simulink library "LibConfigurableSubsystem"  (R2015b)
settings: Solver=VariableStepAuto  StartTime=0.0  StopTime=10.0  RelTol=1e-3
libraries: LibConfigurableSubsystem x1
settings Model: Creator=LUBO  LastModifiedBy=LUBO

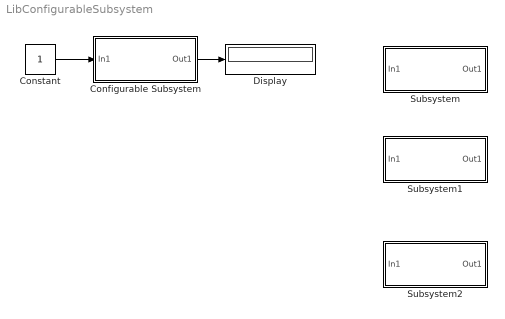
== system LibConfigurableSubsystem ==
  Configurable Subsystem : Subsystem  BlockChoice=Subsystem2
      settings: TemplateBlock=self  MemberBlocks=Subsystem,Subsystem1,Subsystem2
  Constant : Constant
  Display : Display
  Subsystem : Subsystem
  Subsystem1 : Subsystem
  Subsystem2 : Subsystem
  wires:
  Configurable Subsystem/1(Out1) -> Display/1
  Constant/1 -> Configurable Subsystem/1(In1)

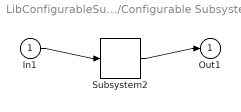
== system LibConfigurableSubsystem/Configurable Subsystem ==
  In1 : Inport
  Subsystem2 : LibConfigurableSubsystem/Subsystem2
  Out1 : Outport
  wires:
  In1/1 -> Subsystem2/1
  Subsystem2/1 -> Out1/1

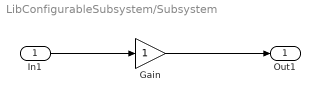
== system LibConfigurableSubsystem/Subsystem ==
  In1 : Inport
  Gain : Gain
  Out1 : Outport
  wires:
  In1/1 -> Gain/1
  Gain/1 -> Out1/1

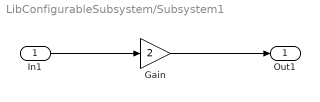
== system LibConfigurableSubsystem/Subsystem1 ==
  In1 : Inport
  Gain : Gain  Gain=2
  Out1 : Outport
  wires:
  In1/1 -> Gain/1
  Gain/1 -> Out1/1

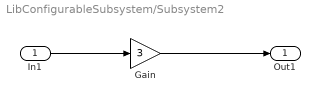
== system LibConfigurableSubsystem/Subsystem2 ==
  In1 : Inport
  Gain : Gain  Gain=3
  Out1 : Outport
  wires:
  In1/1 -> Gain/1
  Gain/1 -> Out1/1
